simulink model "Project1i_haoran9"  (R2021a)
settings: Solver=ode45  StartTime=0.0  StopTime=10  RelTol=1e-3
values from neighbouring files (symbols this model uses):
  ar = -20    [Run_Both_Model.m]    (also in Run_Deadzone.m; Run_Project1i_haoran9.m; Run_ScalarModel.m; Slicing.m)
  astar = -10    [Run_Both_Model.m]    (also in Run_Deadzone.m; Run_Project1i_haoran9.m; Run_ScalarModel.m; Slicing.m)
  br = 20    [Run_Both_Model.m]    (also in Run_Deadzone.m; Run_Project1i_haoran9.m; Run_ScalarModel.m; Slicing.m)
  bstar = +10    (= 10)    [Run_Both_Model.m]    (also in Run_Deadzone.m; Run_Project1i_haoran9.m; Run_ScalarModel.m; Slicing.m)
  gr = 10    [Run_Both_Model.m]    (also in Run_Deadzone.m; Run_Project1i_haoran9.m; Slicing.m; runMatern_MRAC.m)
  gx = 10    [Run_Both_Model.m]    (also in Run_Deadzone.m; Run_Project1i_haoran9.m; Slicing.m; runMatern_MRAC.m)
  kr0 = 0    [Run_Both_Model.m]    (also in Run_Deadzone.m; Run_Project1i_haoran9.m; Run_ScalarModel.m; Slicing.m)
  krstar = br/bstar    (= 2)    [Run_Project1i_haoran9.m]
  kx0 = 0    [Run_Both_Model.m]    (also in Run_Deadzone.m; Run_Project1i_haoran9.m; Run_ScalarModel.m; Slicing.m)
  kxstar = (ar-astar)/bstar    (= -1)    [Run_Project1i_haoran9.m]
  sigma = 0.1    [Run_Both_Model.m]    (also in Run_Deadzone.m; Run_Project1i_haoran9.m; Run_ScalarModel.m; Slicing.m)
  x0 = 0    [Run_Both_Model.m]    (also in Run_Deadzone.m; Run_Project1i_haoran9.m = 1; Run_ScalarModel.m; Slicing.m = 5)
  xr0 = 0    [Run_Both_Model.m]    (also in Run_Deadzone.m; Run_Project1i_haoran9.m; Run_ScalarModel.m; Slicing.m)
settings Model: Creator=owned  LastModifiedBy=Ownedpilot
settings SolverCC: AlgebraicLoopSolver=TrustRegion
settings DebuggingCC: SFMachineParentedDataDiag=warning

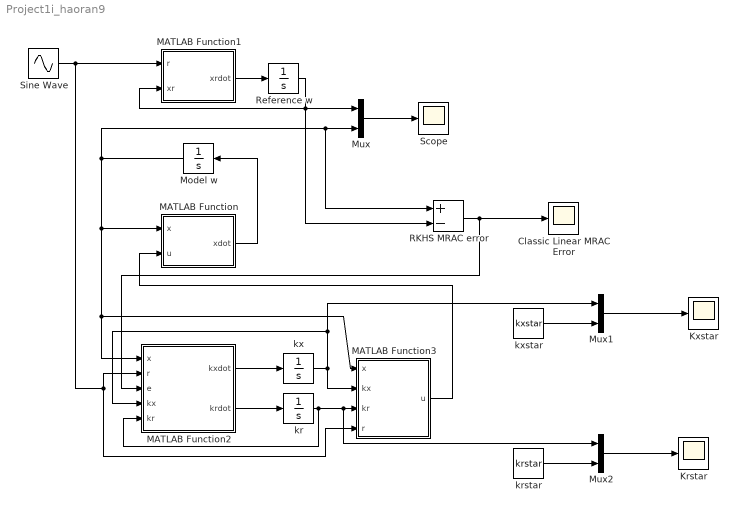
== system Project1i_haoran9 ==
  Classic Linear MRAC Error : Scope
  Krstar : Scope
  Kxstar : Scope
  MATLAB Function : MATLAB Function  TreatAsAtomicUnit=on
  MATLAB Function1 : MATLAB Function  TreatAsAtomicUnit=on
  MATLAB Function2 : MATLAB Function  TreatAsAtomicUnit=on
  MATLAB Function3 : MATLAB Function  TreatAsAtomicUnit=on
  Model w : Integrator  InitialCondition=x0
  Mux : Mux  Inputs=2
  Mux1 : Mux  Inputs=2
  Mux2 : Mux  Inputs=2
  RKHS MRAC error : Sum  Inputs=+-
  Reference w : Integrator  InitialCondition=xr0
  Scope : Scope
  Sine Wave : Sin  Amplitude=10  Frequency=2  SampleTime=0
  kr : Integrator  InitialCondition=kr0
  krstar : Constant  Value=krstar
  kx : Integrator  InitialCondition=kx0
  kxstar : Constant  Value=kxstar
  wires:
  MATLAB Function/1(xdot) -> Model w/1
  Model w/1 -> MATLAB Function/1(x), MATLAB Function3/1(x), MATLAB Function2/1(x), RKHS MRAC error/1, Mux/2
  Sine Wave/1 -> MATLAB Function2/2(r), MATLAB Function3/4(r), MATLAB Function1/1(r)
  MATLAB Function1/1(xrdot) -> Reference w/1
  Reference w/1 -> MATLAB Function1/2(xr), RKHS MRAC error/2, Mux/1
  MATLAB Function2/1(kxdot) -> kx/1
  MATLAB Function2/2(krdot) -> kr/1
  kr/1 -> MATLAB Function2/5(kr), Mux2/1, MATLAB Function3/3(kr)
  kx/1 -> MATLAB Function2/4(kx), Mux1/1, MATLAB Function3/2(kx)
  Mux/1 -> Scope/1
  RKHS MRAC error/1 -> Classic Linear MRAC Error/1, MATLAB Function2/3(e)
  Mux1/1 -> Kxstar/1
  Mux2/1 -> Krstar/1
  kxstar/1 -> Mux1/2
  krstar/1 -> Mux2/2
  MATLAB Function3/1(u) -> MATLAB Function/2(u)

== matlab function Project1i_haoran9/MATLAB Function1 ==
  data: r input; xr input; xrdot output; ar parameter; br parameter
function xrdot = reference(r,xr,ar, br)

xrdot = ar*xr+br*r;

== matlab function Project1i_haoran9/MATLAB Function ==
  data: x input; u input; xdot output; astar parameter; bstar parameter
function xdot = plant(x,u,astar, bstar)

xdot = astar*x+bstar*(u+10*tanh(x));

== matlab function Project1i_haoran9/MATLAB Function2 ==
  data: x input; r input; gx parameter; e input; kxdot output; krdot output; gr parameter; sigma parameter; kx input; kr input
function [kxdot,krdot] = error_dyn(x,r,gx,e, gr,sigma,kx,kr)

kxdot=-gx*x*e-gx*sigma*kx;
krdot=-gr*r*e-gr*sigma*kr;

== matlab function Project1i_haoran9/MATLAB Function3 ==
  data: x input; kx input; u output; kr input; r input
function u = controller(x, kx,kr, r)

u = kx*x+kr*r;
